simulink model "clean_pendulum_math_model"  (R2020b)
settings: Solver=FixedStepAuto  StartTime=0.0  StopTime=200  FixedStep=0.01  RelTol=1e-3
values from neighbouring files (symbols this model uses):
  f_c = 0.5    [clean_pendulum_setup.m]
  f_p = 6.65e-5    (= 6.65e-05)    [clean_pendulum_setup.m]
  g = 9.8101    [Wahadlo_setup.m]    (also in clean_pendulum_setup.m = 9.81)
  I = 1/12 * m_pw * l_c ^ 2      + 1/4 * m_pw * r_c ^ 2      + m_pw * l_c0 ^ 2      + 1/12 * m_ps * l_p ^ 2      + 1/4 * m_pw * r_p ^ 2      + m_ps * l_p0 ^ 2    (= 0.005425772375)    [clean_pendulum_setup.m]
  L = 0.256    [clean_pendulum_setup.m]
  M = 0.503 + 0.045    (= 0.548)    [clean_pendulum_setup.m]
  m = m_c + m_p    (= 63.548)    [Wahadlo_setup.m]    (also in clean_pendulum_setup.m = 0.063)
settings Model: Creator=spika  LastModifiedBy=spika

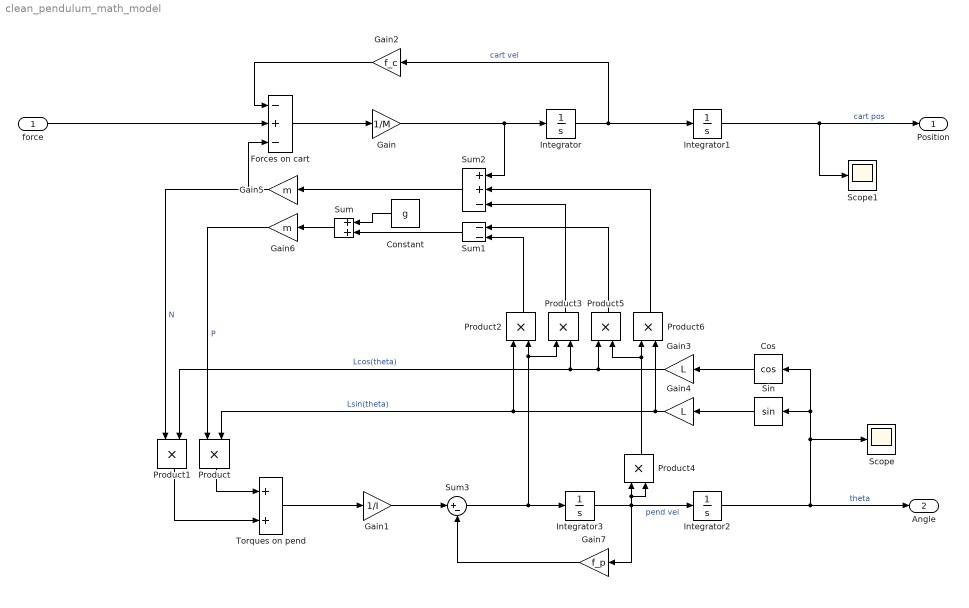
== system clean_pendulum_math_model ==
  force : Inport
  Constant : Constant  Value=g
  Cos : Trigonometry  Operator=cos
  Forces on cart : Sum  Inputs=-+-
  Gain : Gain  Gain=1/M
  Gain1 : Gain  Gain=1/I
  Gain2 : Gain  Gain=f_c
  Gain3 : Gain  Gain=L
  Gain4 : Gain  Gain=L
  Gain5 : Gain  Gain=m
  Gain6 : Gain  Gain=m
  Gain7 : Gain  Gain=f_p
  Integrator : Integrator
  Integrator1 : Integrator
  Integrator2 : Integrator  InitialCondition=pi/2
  Integrator3 : Integrator
  Product{,1..6} (7 alike) : Product
  Scope : Scope
  Scope1 : Scope
  Sin : Trigonometry
  Sum : Sum
  Sum1 : Sum  Inputs=--
  Sum2 : Sum  Inputs=++-
  Sum3 : Sum  Inputs=|+-
  Torques on pend : Sum
  Position : Outport
  Angle : Outport  Port=2
  wires:
  Gain/1 -> Sum2/1, Integrator/1
  Integrator/1 -> Gain2/1, Integrator1/1  "cart vel"
  Integrator1/1 -> Scope1/1, Position/1  "cart pos"
  force/1 -> Forces on cart/2
  Forces on cart/1 -> Gain/1
  Gain2/1 -> Forces on cart/1
  Sum3/1 -> Product3/1, Product2/2, Integrator3/1
  Integrator3/1 -> Gain7/1, Product4/2, Product4/1, Integrator2/1  "pend vel"
  Integrator2/1 -> Scope/1, Cos/1, Sin/1, Angle/1  "theta"
  Torques on pend/1 -> Gain1/1
  Cos/1 -> Gain3/1
  Sin/1 -> Gain4/1
  Gain4/1 -> Product6/2, Product2/1, Product/2  "Lsin(theta)"
  Gain3/1 -> Product5/1, Product3/2, Product1/2  "Lcos(theta)"
  Gain5/1 -> Forces on cart/3, Product1/1  "N"
  Gain6/1 -> Product/1  "P"
  Sum/1 -> Gain6/1
  Constant/1 -> Sum/1
  Sum1/1 -> Sum/2
  Sum2/1 -> Gain5/1
  Product4/1 -> Product5/2, Product6/1
  Product6/1 -> Sum2/2
  Product5/1 -> Sum1/1
  Product3/1 -> Sum2/3
  Product2/1 -> Sum1/2
  Product1/1 -> Torques on pend/2
  Product/1 -> Torques on pend/1
  Gain1/1 -> Sum3/1
  Gain7/1 -> Sum3/2
